simulink model "popul"  (Simulink 8.6)
settings: Solver=FixedStepAuto  StartTime=0.0  StopTime=20  FixedStep=0.0001  RelTol=1e-3
settings Model: Creator=Dinis  LastModifiedBy=Dinis
settings DataIOCC: LimitDataPoints=off  SaveFormat=Dataset  SignalLoggingSaveFormat=Dataset
settings OptimizationCC: ExpressionDepthLimit=128
settings DebuggingCC: UnderspecifiedInitializationDetection=Simplified  MergeDetectMultiDrivingBlocksExec=error  SolverPrmCheckMsg=none  FcnCallInpInsideContextMsg=EnableAllAsError  AllowSymbolicDim=on  StateNameClashWarn=none
settings HardwareCC: ProdBitPerPointer=64  ProdLargestAtomicFloat=Float  ProdIntDivRoundTo=Zero  ProdEndianess=LittleEndian  ProdWordSize=64  ProdHWDeviceType=Intel->x86-64 (Windows64)
settings ModelReferenceCC: PropagateSignalLabelsOutOfModel=on
settings GRTTargetCC: CombineOutputUpdateFcns=on  GRTInterface=off
settings ConfigComp: CovModelRefEnable=off

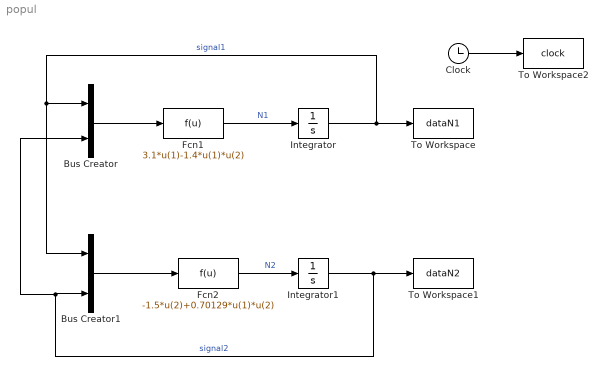
== system popul ==
  Bus Creator : BusCreator  Inputs=2
  Bus Creator1 : BusCreator  Inputs=2
  Clock : Clock
  Fcn1 : Fcn  Expr=3.1*u(1)-1.4*u(1)*u(2)
  Fcn2 : Fcn  Expr=-1.5*u(2)+0.70129*u(1)*u(2)
  Integrator : Integrator  InitialCondition=4
  Integrator1 : Integrator  InitialCondition=1.5982
  To Workspace : ToWorkspace  VariableName=dataN1  SampleTime=-1
  To Workspace1 : ToWorkspace  VariableName=dataN2  SampleTime=-1
  To Workspace2 : ToWorkspace  VariableName=clock  SampleTime=-1
  wires:
  Bus Creator1/1 -> Fcn2/1
  Fcn2/1 -> Integrator1/1  "N2"
  Fcn1/1 -> Integrator/1  "N1"
  Bus Creator/1 -> Fcn1/1
  Integrator/1 -> Bus Creator1/1, Bus Creator/1, To Workspace/1  "signal1"
  Integrator1/1 -> Bus Creator/2, Bus Creator1/2, To Workspace1/1  "signal2"
  Clock/1 -> To Workspace2/1
